simulink model "control_system"  (R2016b)
settings: Solver=VariableStepAuto  StartTime=0.0  StopTime=10.0  RelTol=1e-3
settings Model: Creator=momen  LastModifiedBy=momen

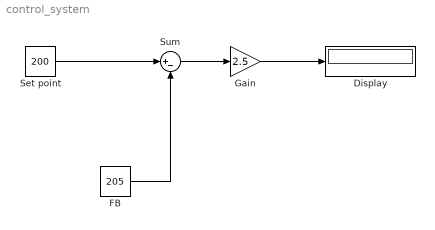
== system control_system ==
  Display : Display
  FB : Constant  Value=205
  Gain : Gain  Gain=2.5
  Set point : Constant  Value=200
  Sum : Sum  Inputs=|+-
  wires:
  FB/1 -> Sum/2
  Set point/1 -> Sum/1
  Sum/1 -> Gain/1
  Gain/1 -> Display/1
